simulink model "eVTOL_Small_nonandlin_algorithm_validation"  (R2024b)
settings: Solver=ode3  StartTime=0.0  StopTime=220  FixedStep=0.02  RelTol=1e-3
undefined symbols (not defined in the file): a_, b, c, c1_, deg, dttrim0, F, g, g1, h1, l1, m, MIL, PARAR, rad, rho, s, T, u_dim, ut, x_dim, xf, xmset, y_dim, yf, ymset, zf, zmset
libraries: simulink x34, aerolibconvert2 x5, aerolibwind2 x2, shared6dof x1
(part 2 of 7)

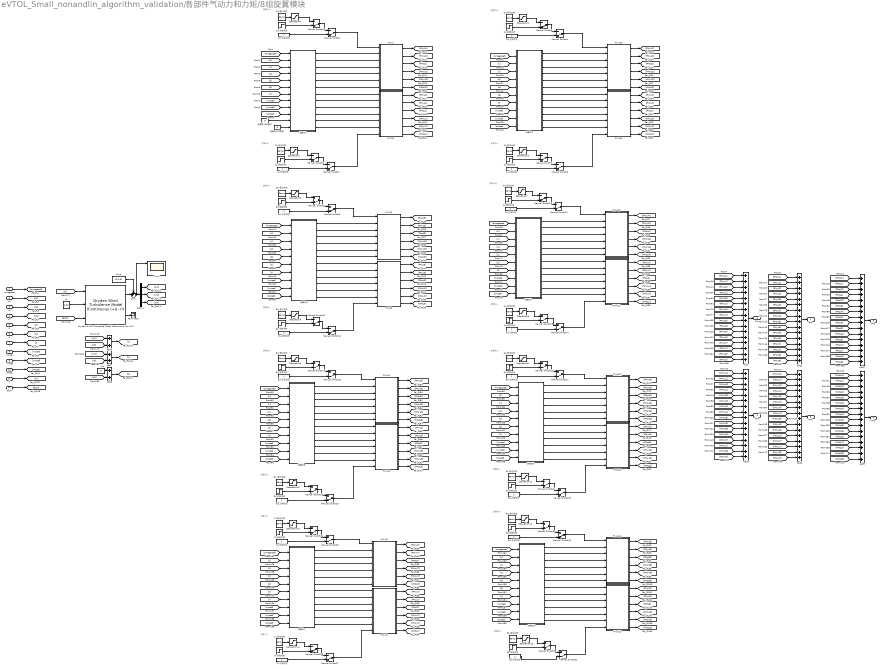
== system eVTOL_Small_nonandlin_algorithm_validation/各部件气动力和力矩/8组旋翼模块 ==
  note: 旋翼4-U
  note: 旋翼2-L
  note: 旋翼6-U
  note: 旋翼6-L
  note: 旋翼7-L
  note: 旋翼5-U
  note: 旋翼4-L
  note: 旋翼7-U
  note: 旋翼3-L
  note: 旋翼3-U
  note: 旋翼5-L
  note: 旋翼2-U
  note: 旋翼1-L
  note: 旋翼1-U
  note: 旋翼8-U
  note: 旋翼8-L
  omegaset : Inport
  u0 : Inport  Port=2
  v0 : Inport  Port=3
  w0 : Inport  Port=4
  p : Inport  Port=5
  q : Inport  Port=6
  r : Inport  Port=7
  xmset : Inport  Port=8
  ymset : Inport  Port=9
  zmset : Inport  Port=10
  H : Inport  Port=11
  DCM : Inport  Port=12
  1L-正常状态 : Constant
  1L-突发失效 : Step  Time=220  Before=1  After=0.5  SampleTime=0
  1L-退化失效 : simulink/Sources/Ramp  slope=0.3325  start=30  InitialOutput=0
  1U-正常状态 : Constant
  1U-突发失效 : Step  Time=140  Before=1  After=0.5  SampleTime=0
  1U-退化失效 : simulink/Sources/Ramp  slope=0.3325  start=30  InitialOutput=0
  2L-正常状态 : Constant
  2L-突发失效 : Step  Time=30  Before=1  After=Lp  SampleTime=0
  2L-退化失效 : simulink/Sources/Ramp  slope=0.3325  start=30  InitialOutput=0
  2U-正常状态 : Constant
  2U-突发失效 : Step  Time=80  Before=1  After=0.6  SampleTime=0
  2U-退化失效 : simulink/Sources/Ramp  slope=0.3325  start=30  InitialOutput=0
  3L-正常状态 : Constant
  3L-突发失效 : Step  Time=30  Before=1  After=Lp  SampleTime=0
  3L-退化失效 : simulink/Sources/Ramp  slope=0.3325  start=30  InitialOutput=0
  3U-正常状态 : Constant
  3U-突发失效 : Step  Time=100  Before=1  After=0.3  SampleTime=0
  3U-退化失效 : simulink/Sources/Ramp  slope=0.3325  start=30  InitialOutput=0
  4L-正常状态 : Constant
  4L-突发失效 : Step  Time=140  Before=1  After=Lp  SampleTime=0
  4L-退化失效 : simulink/Sources/Ramp  slope=0.3325  start=30  InitialOutput=0
  4U-正常状态 : Constant
  4U-突发失效 : Step  Time=160  Before=1  After=0.7  SampleTime=0
  4U-退化失效 : simulink/Sources/Ramp  slope=0.3325  start=30  InitialOutput=0
  5L -退化失效 : simulink/Sources/Ramp  slope=0.3325  start=30  InitialOutput=0
  5L-正常状态 : Constant
  5L-突发失效 : Step  Time=100  Before=1  After=Lp  SampleTime=0
  5U-正常状态 : Constant
  5U-突发失效 : Step  Time=60  Before=1  After=0.4  SampleTime=0
  5U-退化失效 : simulink/Sources/Ramp  slope=0.3325  start=30  InitialOutput=0
  6L-正常状态 : Constant
  6L-突发失效 : Step  Time=30  Before=1  After=Lp  SampleTime=0
  6L-退化失效 : simulink/Sources/Ramp  slope=0.3325  start=30  InitialOutput=0
  6U-正常状态 : Constant
  6U-突发失效 : Step  Time=160  Before=1  After=0.8  SampleTime=0
  6U-退化失效 : simulink/Sources/Ramp  slope=0.3325  start=30  InitialOutput=0
  7L-正常状态 : Constant
  7L-突发失效 : Step  Time=220  Before=1  After=0.5  SampleTime=0
  7L-退化失效 : simulink/Sources/Ramp  slope=0.3325  start=30  InitialOutput=0
  7U-正常状态 : Constant
  7U-突发失效 : Step  Time=80  Before=1  After=0.6  SampleTime=0
  7U-退化失效 : simulink/Sources/Ramp  slope=0.3325  start=30  InitialOutput=0
  8L-正常状态 : Constant
  8L-突发失效 : Step  Time=180  Before=1  After=Lp  SampleTime=0
  8L-退化失效 : simulink/Sources/Ramp  slope=0.3325  start=30  InitialOutput=0
  8U-正常状态 : Constant
  8U-突发失效 : Step  Time=180  Before=1  After=0.5  SampleTime=0
  8U-退化失效 : simulink/Sources/Ramp  slope=0.3325  start=30  InitialOutput=0
  Add{,1..5} (6 alike) : Sum  Inputs=++++++++++++++++
  Add6 : Sum
  Add7 : Sum
  Add8 : Sum
  Demux : Demux  Outputs=3
  Dryden Wind Turbulence Model (Continuous (+q +r))1 : aerolibwind2/Dryden Wind Turbulence Model  (Continuous (+q -r))  units=Metric (MKS)  spec=MIL-F-8785C  model=Continuous Dryden (+q +r)  W20=10  Wdeg=45  TurbProb=2x10^-1  L_high=1  Wingspan=1  ts=0.1  Seed=[23341 23342 23343 23344]  T_on=on
  FI-1-U : Subsystem
  FI-1-U1 : Subsystem
  FI-1-U10 : Subsystem
  FI-1-U11 : Subsystem
  FI-1-U12 : Subsystem
  FI-1-U13 : Subsystem
  FI-1-U14 : Subsystem
  FI-1-U15 : Subsystem
  FI-1-U2 : Subsystem
  FI-1-U3 : Subsystem
  FI-1-U4 : Subsystem
  FI-1-U5 : Subsystem
  FI-1-U6 : Subsystem
  FI-1-U7 : Subsystem
  FI-1-U8 : Subsystem
  FI-1-U9 : Subsystem
  Manual Switch{1..32} (32 alike) : ManualSwitch  CurrentSetting=0
  Saturation{1..16} (16 alike) : Saturate  UpperLimit=10  LowerLimit=0
  Sum : Sum  Inputs=++|
  T+W : Scope  NumInputPorts=3
  Terminator : Terminator
  Vs : Constant  Value=0.01
  Wind : Constant  Value=[0,0,0]
  wW : Constant  Value=0
  旋翼组1 : Subsystem
  旋翼组2 : Subsystem
  旋翼组3 : Subsystem
  旋翼组4 : Subsystem
  旋翼组5 : Subsystem
  旋翼组6 : Subsystem
  旋翼组7 : Subsystem
  旋翼组8 : Subsystem
  旋翼轴1前倾角° : Constant  Value=0
  旋翼轴1右倾角° : Constant  Value=0
  FMx : Outport  VectorParamsAs1DForOutWhenUnconnected=off
  FMy : Outport  Port=2  VectorParamsAs1DForOutWhenUnconnected=off
  FMz : Outport  Port=3  VectorParamsAs1DForOutWhenUnconnected=off
  MMx : Outport  Port=4  VectorParamsAs1DForOutWhenUnconnected=off
  MMy : Outport  Port=5  VectorParamsAs1DForOutWhenUnconnected=off
  MMz : Outport  Port=6  VectorParamsAs1DForOutWhenUnconnected=off
  wires:
  omegaset/1 -> [omegaset]
  u0/1 -> [u0]
  v0/1 -> [v0]
  w0/1 -> [w0]
  p/1 -> [p]
  r/1 -> [r]
  q/1 -> [q]
  xmset/1 -> [xmset]
  ymset/1 -> [ymset]
  zmset/1 -> [zmset]
  H/1 -> [H]
  DCM/1 -> [DCM]
  [v0] -> Add7/2
  [vW] -> Add7/1
  Add7/1 -> [v]
  Add6/1 -> [u]
  Demux/2 -> [vW]
  [u0] -> Add6/2
  Vs/1 -> Dryden Wind Turbulence Model (Continuous (+q +r))1/2
  Dryden Wind Turbulence Model (Continuous (+q +r))1/2 -> Terminator/1
  [uW] -> Add6/1
  Add8/1 -> [w]
  wW/1 -> Add8/1
  [w0] -> Add8/2
  Demux/3 -> [wW]
  [H] -> Dryden Wind Turbulence Model (Continuous (+q +r))1/1
  Demux/1 -> [uW]
  [DCM] -> Dryden Wind Turbulence Model (Continuous (+q +r))1/3
  [FMyL5] -> Add1/10
  [MMyU7] -> Add4/13
  [MMzU4] -> Add5/7
  [FMzU3] -> Add2/5
  [MMxU5] -> Add3/9
  [MMxL2] -> Add3/4
  [MMzU3] -> Add5/5
  [MMyU4] -> Add4/7
  [MMxU4] -> Add3/7
  旋翼轴1右倾角°/1 -> 旋翼组1/12(ILR)
  [MMzL4] -> Add5/8
  [FMyU5] -> Add1/9
  [MMxL6] -> Add3/12
  [v] -> 旋翼组2/3(v)
  [MMyL1] -> Add4/2
  [MMzU6] -> Add5/11
  [FMxU7] -> Add/13
  [FMxL6] -> Add/12
  [MMzL2] -> Add5/4
  旋翼轴1前倾角°/1 -> 旋翼组1/11(ISR)
  [MMxL5] -> Add3/10
  [MMyL5] -> Add4/10
  [FMzL7] -> Add2/14
  [omegaset] -> 旋翼组1/1(omegaset)
  [FMzU1] -> Add2/1
  [MMyU1] -> Add4/1
  [MMzU1] -> Add5/1
  [FMyL1] -> Add1/2
  [MMyU2] -> Add4/3
  [MMyU3] -> Add4/5
  [FMyU4] -> Add1/7
  [FMzL5] -> Add2/10
  [MMyU6] -> Add4/11
  [FMxL7] -> Add/14
  [MMyL6] -> Add4/12
  [FMzU6] -> Add2/11
  [FMyU1] -> Add1/1
  [zmset] -> 旋翼组1/10(zmset)
  [q] -> 旋翼组1/6(q)
  [u] -> 旋翼组1/2(u)
  [w] -> 旋翼组1/4(w)
  [FMyU6] -> Add1/11
  [MMxL3] -> Add3/6
  [p] -> 旋翼组1/5(p)
  [FMxU5] -> Add/9
  [v] -> 旋翼组1/3(v)
  [FMxL4] -> Add/8
  Add1/1 -> FMy/1
  [FMyU7] -> Add1/13
  [MMzL6] -> Add5/12
  [FMyL7] -> Add1/14
  [FMzU5] -> Add2/9
  [MMxU3] -> Add3/5
  [MMzU2] -> Add5/3
  [xmset] -> 旋翼组1/8(xmset)
  [MMyL4] -> Add4/8
  [ymset] -> 旋翼组2/9(ymset)
  [MMxL4] -> Add3/8
  [MMxU6] -> Add3/11
  [u] -> 旋翼组2/2(u)
  [MMyU5] -> Add4/9
  [omegaset] -> 旋翼组2/1(omegaset)
  [FMxU2] -> Add/3
  [q] -> 旋翼组2/6(q)
  [FMxL5] -> Add/10
  [w] -> 旋翼组2/4(w)
  [FMyL6] -> Add1/12
  [p] -> 旋翼组2/5(p)
  [FMxL8] -> Add/16
  [ymset] -> 旋翼组1/9(ymset)
  [r] -> 旋翼组1/7(r)
  Add2/1 -> FMz/1
  [FMzL6] -> Add2/12
  [FMxU8] -> Add/15
  [FMyU8] -> Add1/15
  [MMxU7] -> Add3/13
  [MMxU8] -> Add3/15
  [FMxL1] -> Add/2
  [xmset] -> 旋翼组2/8(xmset)
  [FMzU8] -> Add2/15
  [MMyL2] -> Add4/4
  [FMxU3] -> Add/5
  [zmset] -> 旋翼组2/10(zmset)
  [MMzL1] -> Add5/2
  [MMyL3] -> Add4/6
  [MMzU7] -> Add5/13
  [MMyU8] -> Add4/15
  [FMzU2] -> Add2/3
  [MMzL5] -> Add5/10
  [FMyL8] -> Add1/16
  [FMxU1] -> Add/1
  Add5/1 -> MMz/1
  Add4/1 -> MMy/1
  [MMyL7] -> Add4/14
  [MMxL1] -> Add3/2
  [MMzL7] -> Add5/14
  [MMzU5] -> Add5/9
  [FMzL2] -> Add2/4
  [FMyL2] -> Add1/4
  [MMxL8] -> Add3/16
  [FMzL4] -> Add2/8
  [MMzL3] -> Add5/6
  [MMxL7] -> Add3/14
  [MMxU1] -> Add3/1
  [FMzL3] -> Add2/6
  Add3/1 -> MMx/1
  [r] -> 旋翼组2/7(r)
  [FMyL4] -> Add1/8
  [MMyL8] -> Add4/16
  [MMxU2] -> Add3/3
  [FMzU7] -> Add2/13
  [FMxL2] -> Add/4
  [FMyU3] -> Add1/5
  [FMzL8] -> Add2/16
  Add/1 -> FMx/1
  [FMzU4] -> Add2/7
  [FMzL1] -> Add2/2
  [FMxL3] -> Add/6
  [FMyU2] -> Add1/3
  [FMxU4] -> Add/7
  [FMyL3] -> Add1/6
  [MMzU8] -> Add5/15
  [MMzL8] -> Add5/16
  [FMxU6] -> Add/11
  Sum/1 -> T+W/1, Demux/1
  Wind/1 -> Sum/1
  [zmset] -> 旋翼组6/10(zmset)
  [r] -> 旋翼组5/7(r)
  [omegaset] -> 旋翼组4/1(omegaset)
  [p] -> 旋翼组7/5(p)
  [ymset] -> 旋翼组7/9(ymset)
  [p] -> 旋翼组4/5(p)
  [omegaset] -> 旋翼组7/1(omegaset)
  [xmset] -> 旋翼组6/8(xmset)
  [w] -> 旋翼组6/4(w)
  [q] -> 旋翼组6/6(q)
  [xmset] -> 旋翼组7/8(xmset)
  [zmset] -> 旋翼组8/10(zmset)
  [omegaset] -> 旋翼组6/1(omegaset)
  [v] -> 旋翼组5/3(v)
  [v] -> 旋翼组6/3(v)
  [q] -> 旋翼组7/6(q)
  [p] -> 旋翼组6/5(p)
  [ymset] -> 旋翼组8/9(ymset)
  [r] -> 旋翼组7/7(r)
  [p] -> 旋翼组8/5(p)
  [xmset] -> 旋翼组4/8(xmset)
  [w] -> 旋翼组4/4(w)
  [u] -> 旋翼组8/2(u)
  [q] -> 旋翼组4/6(q)
  [omegaset] -> 旋翼组8/1(omegaset)
  [u] -> 旋翼组6/2(u)
  [zmset] -> 旋翼组3/10(zmset)
  [ymset] -> 旋翼组5/9(ymset)
  [u] -> 旋翼组3/2(u)
  [u] -> 旋翼组4/2(u)
  [r] -> 旋翼组6/7(r)
  [w] -> 旋翼组3/4(w)
  [zmset] -> 旋翼组4/10(zmset)
  [q] -> 旋翼组3/6(q)
  [ymset] -> 旋翼组4/9(ymset)
  [xmset] -> 旋翼组3/8(xmset)
  [p] -> 旋翼组3/5(p)
  [r] -> 旋翼组8/7(r)
  [v] -> 旋翼组8/3(v)
  [q] -> 旋翼组5/6(q)
  [p] -> 旋翼组5/5(p)
  [ymset] -> 旋翼组3/9(ymset)
  [r] -> 旋翼组3/7(r)
  [u] -> 旋翼组5/2(u)
  [r] -> 旋翼组4/7(r)
  [v] -> 旋翼组4/3(v)
  [v] -> 旋翼组7/3(v)
  [ymset] -> 旋翼组6/9(ymset)
  [xmset] -> 旋翼组5/8(xmset)
  [w] -> 旋翼组7/4(w)
  [xmset] -> 旋翼组8/8(xmset)
  [v] -> 旋翼组3/3(v)
  [q] -> 旋翼组8/6(q)
  [zmset] -> 旋翼组7/10(zmset)
  [w] -> 旋翼组8/4(w)
  [u] -> 旋翼组7/2(u)
  [zmset] -> 旋翼组5/10(zmset)
  [w] -> 旋翼组5/4(w)
  [omegaset] -> 旋翼组3/1(omegaset)
  [omegaset] -> 旋翼组5/1(omegaset)
  Dryden Wind Turbulence Model (Continuous (+q +r))1/1 -> Sum/2
  旋翼组1/1(FMxU1) -> FI-1-U/2(FMxU1)
  旋翼组1/2(FMyU1) -> FI-1-U/3(FMyU1)
  旋翼组1/3(FMzU1) -> FI-1-U/4(FMzU1)
  旋翼组1/4(MMxU1) -> FI-1-U/5(MMxU1)
  旋翼组1/5(MMyU1) -> FI-1-U/6(MMyU1)
  旋翼组1/6(MMzU1) -> FI-1-U/7(MMzU1)
  FI-1-U/6(Out6) -> [MMzU1]
  FI-1-U/5(Out5) -> [MMyU1]
  FI-1-U/4(Out4) -> [MMxU1]
  FI-1-U/3(Out3) -> [FMzU1]
  FI-1-U/2(Out2) -> [FMyU1]
  FI-1-U/1(Out1) -> [FMxU1]
  FI-1-U2/3(Out3) -> [FMzU3]
  FI-1-U2/6(Out6) -> [MMzU3]
  FI-1-U2/1(Out1) -> [FMxU3]
  FI-1-U3/1(Out1) -> [FMxL3]
  FI-1-U2/2(Out2) -> [FMyU3]
  FI-1-U3/2(Out2) -> [FMyL3]
  FI-1-U2/5(Out5) -> [MMyU3]
  FI-1-U2/4(Out4) -> [MMxU3]
  FI-1-U3/4(Out4) -> [MMxL3]
  FI-1-U3/5(Out5) -> [MMyL3]
  FI-1-U3/3(Out3) -> [FMzL3]
  5U-突发失效/1 -> Manual Switch17/2
  3L-退化失效/1 -> Saturation6/1
  Manual Switch11/1 -> Manual Switch10/1
  6U-正常状态/1 -> Manual Switch21/2
  3L-正常状态/1 -> Manual Switch10/2
  1U-突发失效/1 -> Manual Switch20/2
  4U-正常状态/1 -> Manual Switch12/2
  2U-正常状态/1 -> Manual Switch4/2
  5L-正常状态/1 -> Manual Switch18/2
  Saturation12/1 -> Manual Switch24/1
  7U-退化失效/1 -> Saturation13/1
  Saturation6/1 -> Manual Switch11/1
  4L-退化失效/1 -> Saturation8/1
  Manual Switch20/1 -> Manual Switch1/1
  4L-突发失效/1 -> Manual Switch15/2
  Saturation14/1 -> Manual Switch28/1
  7L-退化失效/1 -> Saturation14/1
  6L-退化失效/1 -> Saturation12/1
  4U-退化失效/1 -> Saturation7/1
  6U-突发失效/1 -> Manual Switch22/2
  Saturation10/1 -> Manual Switch19/1
  Manual Switch28/1 -> Manual Switch27/1
  6L-突发失效/1 -> Manual Switch24/2
  4U-突发失效/1 -> Manual Switch13/2
  Saturation7/1 -> Manual Switch13/1
  Manual Switch13/1 -> Manual Switch12/1
  Manual Switch7/1 -> Manual Switch6/1
  1L-突发失效/1 -> Manual Switch3/2
  7L-正常状态/1 -> Manual Switch27/2
  Saturation13/1 -> Manual Switch26/1
  1L-正常状态/1 -> Manual Switch2/2
  Manual Switch26/1 -> Manual Switch25/1
  1U-退化失效/1 -> Saturation4/1
  Manual Switch9/1 -> Manual Switch8/1
  Manual Switch3/1 -> Manual Switch2/1
  Manual Switch5/1 -> Manual Switch4/1
  2U-突发失效/1 -> Manual Switch5/2
  Manual Switch22/1 -> Manual Switch21/1
  2U-退化失效/1 -> Saturation2/1
  1U-正常状态/1 -> Manual Switch1/2
  Saturation2/1 -> Manual Switch5/1
  2L-突发失效/1 -> Manual Switch7/2
  3U-突发失效/1 -> Manual Switch9/2
  Manual Switch15/1 -> Manual Switch14/1
  4L-正常状态/1 -> Manual Switch14/2
  Saturation8/1 -> Manual Switch15/1
  3U-正常状态/1 -> Manual Switch8/2
  Manual Switch17/1 -> Manual Switch16/1
  5U-退化失效/1 -> Saturation9/1
  1L-退化失效/1 -> Saturation1/1
  5U-正常状态/1 -> Manual Switch16/2
  5L -退化失效/1 -> Saturation10/1
  2L-退化失效/1 -> Saturation3/1
  Saturation11/1 -> Manual Switch22/1
  Manual Switch19/1 -> Manual Switch18/1
  Saturation9/1 -> Manual Switch17/1
  2L-正常状态/1 -> Manual Switch6/2
  Saturation3/1 -> Manual Switch7/1
  Saturation5/1 -> Manual Switch9/1
  6U-退化失效/1 -> Saturation11/1
  Manual Switch24/1 -> Manual Switch23/1
  3L-突发失效/1 -> Manual Switch11/2
  7U-突发失效/1 -> Manual Switch26/2
  5L-突发失效/1 -> Manual Switch19/2
  6L-正常状态/1 -> Manual Switch23/2
  Saturation1/1 -> Manual Switch3/1
  3U-退化失效/1 -> Saturation5/1
  Saturation4/1 -> Manual Switch20/1
  7U-正常状态/1 -> Manual Switch25/2
  7L-突发失效/1 -> Manual Switch28/2
  Manual Switch1/1 -> FI-1-U/1(Fault inject)
  旋翼组1/7(FMxL1) -> FI-1-U1/1(FMxU1)
  旋翼组1/8(FMyL1) -> FI-1-U1/2(FMyU1)
  旋翼组1/9(FMzL1) -> FI-1-U1/3(FMzU1)
  旋翼组1/10(MMxL1) -> FI-1-U1/4(MMxU1)
  旋翼组1/11(MMyL1) -> FI-1-U1/5(MMyU1)
  旋翼组1/12(MMzL1) -> FI-1-U1/6(MMzU1)
  FI-1-U1/1(Out1) -> [FMxL1]
  FI-1-U1/2(Out2) -> [FMyL1]
  FI-1-U1/3(Out3) -> [FMzL1]
  FI-1-U1/4(Out4) -> [MMxL1]
  FI-1-U1/5(Out5) -> [MMyL1]
  FI-1-U1/6(Out6) -> [MMzL1]
  Manual Switch2/1 -> FI-1-U1/7(Fault inject)
  旋翼组3/5(MMyU3) -> FI-1-U2/6(MMyU1)
  旋翼组3/6(MMzU3) -> FI-1-U2/7(MMzU1)
  Manual Switch8/1 -> FI-1-U2/1(Fault inject)
  旋翼组3/7(FMxL3) -> FI-1-U3/1(FMxU1)
  旋翼组3/10(MMxL3) -> FI-1-U3/4(MMxU1)
  旋翼组3/1(FMxU3) -> FI-1-U2/2(FMxU1)
  旋翼组3/9(FMzL3) -> FI-1-U3/3(FMzU1)
  旋翼组3/4(MMxU3) -> FI-1-U2/5(MMxU1)
  旋翼组3/12(MMzL3) -> FI-1-U3/6(MMzU1)
  旋翼组3/2(FMyU3) -> FI-1-U2/3(FMyU1)
  Manual Switch10/1 -> FI-1-U3/7(Fault inject)
  旋翼组3/8(FMyL3) -> FI-1-U3/2(FMyU1)
  旋翼组3/3(FMzU3) -> FI-1-U2/4(FMzU1)
  旋翼组3/11(MMyL3) -> FI-1-U3/5(MMyU1)
  FI-1-U3/6(Out6) -> [MMzL3]
  FI-1-U5/6(Out6) -> [MMzL5]
  旋翼组5/11(MMyL5) -> FI-1-U5/5(MMyU1)
  旋翼组5/3(FMzU5) -> FI-1-U4/4(FMzU1)
  Manual Switch16/1 -> FI-1-U4/1(Fault inject)
  旋翼组5/10(MMxL5) -> FI-1-U5/4(MMxU1)
  FI-1-U4/2(Out2) -> [FMyU5]
  FI-1-U4/5(Out5) -> [MMyU5]
  旋翼组5/7(FMxL5) -> FI-1-U5/1(FMxU1)
  旋翼组5/5(MMyU5) -> FI-1-U4/6(MMyU1)
  旋翼组5/8(FMyL5) -> FI-1-U5/2(FMyU1)
  旋翼组5/9(FMzL5) -> FI-1-U5/3(FMzU1)
  Manual Switch18/1 -> FI-1-U5/7(Fault inject)
  FI-1-U4/6(Out6) -> [MMzU5]
  旋翼组5/2(FMyU5) -> FI-1-U4/3(FMyU1)
  FI-1-U5/4(Out4) -> [MMxL5]
  旋翼组5/4(MMxU5) -> FI-1-U4/5(MMxU1)
  旋翼组5/6(MMzU5) -> FI-1-U4/7(MMzU1)
  FI-1-U4/1(Out1) -> [FMxU5]
  FI-1-U4/3(Out3) -> [FMzU5]
  FI-1-U5/3(Out3) -> [FMzL5]
  旋翼组5/12(MMzL5) -> FI-1-U5/6(MMzU1)
  旋翼组5/1(FMxU5) -> FI-1-U4/2(FMxU1)
  FI-1-U5/5(Out5) -> [MMyL5]
  FI-1-U5/1(Out1) -> [FMxL5]
  FI-1-U5/2(Out2) -> [FMyL5]
  FI-1-U4/4(Out4) -> [MMxU5]
  旋翼组7/7(FMxL7) -> FI-1-U7/1(FMxU1)
  旋翼组7/4(MMxU7) -> FI-1-U6/5(MMxU1)
  Manual Switch27/1 -> FI-1-U7/7(Fault inject)
  旋翼组7/1(FMxU7) -> FI-1-U6/2(FMxU1)
  Manual Switch25/1 -> FI-1-U6/1(Fault inject)
  旋翼组7/8(FMyL7) -> FI-1-U7/2(FMyU1)
  旋翼组7/11(MMyL7) -> FI-1-U7/5(MMyU1)
  旋翼组7/9(FMzL7) -> FI-1-U7/3(FMzU1)
  旋翼组7/10(MMxL7) -> FI-1-U7/4(MMxU1)
  FI-1-U6/2(Out2) -> [FMyU7]
  旋翼组7/3(FMzU7) -> FI-1-U6/4(FMzU1)
  旋翼组7/6(MMzU7) -> FI-1-U6/7(MMzU1)
  旋翼组7/5(MMyU7) -> FI-1-U6/6(MMyU1)
  FI-1-U6/6(Out6) -> [MMzU7]
  旋翼组7/12(MMzL7) -> FI-1-U7/6(MMzU1)
  FI-1-U7/6(Out6) -> [MMzL7]
  旋翼组7/2(FMyU7) -> FI-1-U6/3(FMyU1)
  FI-1-U6/3(Out3) -> [FMzU7]
  FI-1-U6/4(Out4) -> [MMxU7]
  FI-1-U7/1(Out1) -> [FMxL7]
  FI-1-U6/5(Out5) -> [MMyU7]
  FI-1-U7/2(Out2) -> [FMyL7]
  FI-1-U7/5(Out5) -> [MMyL7]
  FI-1-U6/1(Out1) -> [FMxU7]
  FI-1-U7/3(Out3) -> [FMzL7]
  FI-1-U7/4(Out4) -> [MMxL7]
  旋翼组2/4(MMxU2) -> FI-1-U8/5(MMxU1)
  FI-1-U8/1(Out1) -> [FMxU2]
  FI-1-U8/6(Out6) -> [MMzU2]
  FI-1-U9/5(Out5) -> [MMyL2]
  FI-1-U9/2(Out2) -> [FMyL2]
  Manual Switch4/1 -> FI-1-U8/1(Fault inject)
  旋翼组2/2(FMyU2) -> FI-1-U8/3(FMyU1)
  旋翼组2/7(FMxL2) -> FI-1-U9/1(FMxU1)
  旋翼组2/10(MMxL2) -> FI-1-U9/4(MMxU1)
  FI-1-U8/2(Out2) -> [FMyU2]
  FI-1-U8/4(Out4) -> [MMxU2]
  FI-1-U9/4(Out4) -> [MMxL2]
  旋翼组2/3(FMzU2) -> FI-1-U8/4(FMzU1)
  旋翼组2/5(MMyU2) -> FI-1-U8/6(MMyU1)
  旋翼组2/1(FMxU2) -> FI-1-U8/2(FMxU1)
  旋翼组2/9(FMzL2) -> FI-1-U9/3(FMzU1)
  旋翼组2/8(FMyL2) -> FI-1-U9/2(FMyU1)
  旋翼组2/6(MMzU2) -> FI-1-U8/7(MMzU1)
  FI-1-U8/5(Out5) -> [MMyU2]
  旋翼组2/11(MMyL2) -> FI-1-U9/5(MMyU1)
  旋翼组2/12(MMzL2) -> FI-1-U9/6(MMzU1)
  FI-1-U8/3(Out3) -> [FMzU2]
  FI-1-U9/1(Out1) -> [FMxL2]
  FI-1-U9/6(Out6) -> [MMzL2]
  FI-1-U9/3(Out3) -> [FMzL2]
  Manual Switch6/1 -> FI-1-U9/7(Fault inject)
  旋翼组4/2(FMyU4) -> FI-1-U10/3(FMyU1)
  旋翼组4/11(MMyL4) -> FI-1-U11/5(MMyU1)
  旋翼组4/6(MMzU4) -> FI-1-U10/7(MMzU1)
  旋翼组4/4(MMxU4) -> FI-1-U10/5(MMxU1)
  FI-1-U10/3(Out3) -> [FMzU4]
  FI-1-U11/6(Out6) -> [MMzL4]
  旋翼组4/9(FMzL4) -> FI-1-U11/3(FMzU1)
  旋翼组4/3(FMzU4) -> FI-1-U10/4(FMzU1)
  旋翼组4/7(FMxL4) -> FI-1-U11/1(FMxU1)
  旋翼组4/12(MMzL4) -> FI-1-U11/6(MMzU1)
  旋翼组4/1(FMxU4) -> FI-1-U10/2(FMxU1)
  FI-1-U10/4(Out4) -> [MMxU4]
  旋翼组4/5(MMyU4) -> FI-1-U10/6(MMyU1)
  旋翼组4/10(MMxL4) -> FI-1-U11/4(MMxU1)
  旋翼组4/8(FMyL4) -> FI-1-U11/2(FMyU1)
  Manual Switch14/1 -> FI-1-U11/7(Fault inject)
  Manual Switch12/1 -> FI-1-U10/1(Fault inject)
  FI-1-U10/6(Out6) -> [MMzU4]
  FI-1-U11/2(Out2) -> [FMyL4]
  FI-1-U10/5(Out5) -> [MMyU4]
  FI-1-U10/2(Out2) -> [FMyU4]
  FI-1-U10/1(Out1) -> [FMxU4]
  FI-1-U11/5(Out5) -> [MMyL4]
  FI-1-U11/4(Out4) -> [MMxL4]
  FI-1-U11/3(Out3) -> [FMzL4]
  FI-1-U11/1(Out1) -> [FMxL4]
  旋翼组6/9(FMzL6) -> FI-1-U13/3(FMzU1)
  旋翼组6/4(MMxU6) -> FI-1-U12/5(MMxU1)
  FI-1-U12/1(Out1) -> [FMxU6]
  FI-1-U12/2(Out2) -> [FMyU6]
  FI-1-U13/4(Out4) -> [MMxL6]
  FI-1-U13/2(Out2) -> [FMyL6]
  Manual Switch21/1 -> FI-1-U12/1(Fault inject)
  旋翼组6/5(MMyU6) -> FI-1-U12/6(MMyU1)
  FI-1-U12/6(Out6) -> [MMzU6]
  旋翼组6/1(FMxU6) -> FI-1-U12/2(FMxU1)
  旋翼组6/12(MMzL6) -> FI-1-U13/6(MMzU1)
  旋翼组6/2(FMyU6) -> FI-1-U12/3(FMyU1)
  FI-1-U13/6(Out6) -> [MMzL6]
  旋翼组6/6(MMzU6) -> FI-1-U12/7(MMzU1)
  旋翼组6/11(MMyL6) -> FI-1-U13/5(MMyU1)
  FI-1-U12/3(Out3) -> [FMzU6]
  旋翼组6/3(FMzU6) -> FI-1-U12/4(FMzU1)
  旋翼组6/8(FMyL6) -> FI-1-U13/2(FMyU1)
  旋翼组6/7(FMxL6) -> FI-1-U13/1(FMxU1)
  FI-1-U13/1(Out1) -> [FMxL6]
  FI-1-U12/5(Out5) -> [MMyU6]
  FI-1-U12/4(Out4) -> [MMxU6]
  旋翼组6/10(MMxL6) -> FI-1-U13/4(MMxU1)
  Manual Switch23/1 -> FI-1-U13/7(Fault inject)
  FI-1-U13/3(Out3) -> [FMzL6]
  FI-1-U13/5(Out5) -> [MMyL6]
  旋翼组8/10(MMxL8) -> FI-1-U15/4(MMxU1)
  旋翼组8/4(MMxU8) -> FI-1-U14/5(MMxU1)
  FI-1-U15/4(Out4) -> [MMxL8]
  FI-1-U15/6(Out6) -> [MMzL8]
  FI-1-U14/6(Out6) -> [MMzU8]
  FI-1-U15/3(Out3) -> [FMzL8]
  Manual Switch29/1 -> FI-1-U14/1(Fault inject)
  FI-1-U14/2(Out2) -> [FMyU8]
  Manual Switch31/1 -> FI-1-U15/7(Fault inject)
  旋翼组8/5(MMyU8) -> FI-1-U14/6(MMyU1)
  旋翼组8/3(FMzU8) -> FI-1-U14/4(FMzU1)
  旋翼组8/6(MMzU8) -> FI-1-U14/7(MMzU1)
  旋翼组8/1(FMxU8) -> FI-1-U14/2(FMxU1)
  FI-1-U14/4(Out4) -> [MMxU8]
  FI-1-U14/5(Out5) -> [MMyU8]
  旋翼组8/9(FMzL8) -> FI-1-U15/3(FMzU1)
  旋翼组8/2(FMyU8) -> FI-1-U14/3(FMyU1)
  FI-1-U15/1(Out1) -> [FMxL8]
  FI-1-U14/1(Out1) -> [FMxU8]
  FI-1-U14/3(Out3) -> [FMzU8]
  旋翼组8/11(MMyL8) -> FI-1-U15/5(MMyU1)
  旋翼组8/12(MMzL8) -> FI-1-U15/6(MMzU1)
  旋翼组8/7(FMxL8) -> FI-1-U15/1(FMxU1)
  旋翼组8/8(FMyL8) -> FI-1-U15/2(FMyU1)
  FI-1-U15/2(Out2) -> [FMyL8]
  Manual Switch30/1 -> Manual Switch29/1
  8U-退化失效/1 -> Saturation15/1
  Manual Switch32/1 -> Manual Switch31/1
  8L-正常状态/1 -> Manual Switch31/2
  8L-退化失效/1 -> Saturation16/1
  8L-突发失效/1 -> Manual Switch32/2
  8U-突发失效/1 -> Manual Switch30/2
  8U-正常状态/1 -> Manual Switch29/2
  Saturation16/1 -> Manual Switch32/1
  Saturation15/1 -> Manual Switch30/1
  FI-1-U15/5(Out5) -> [MMyL8]

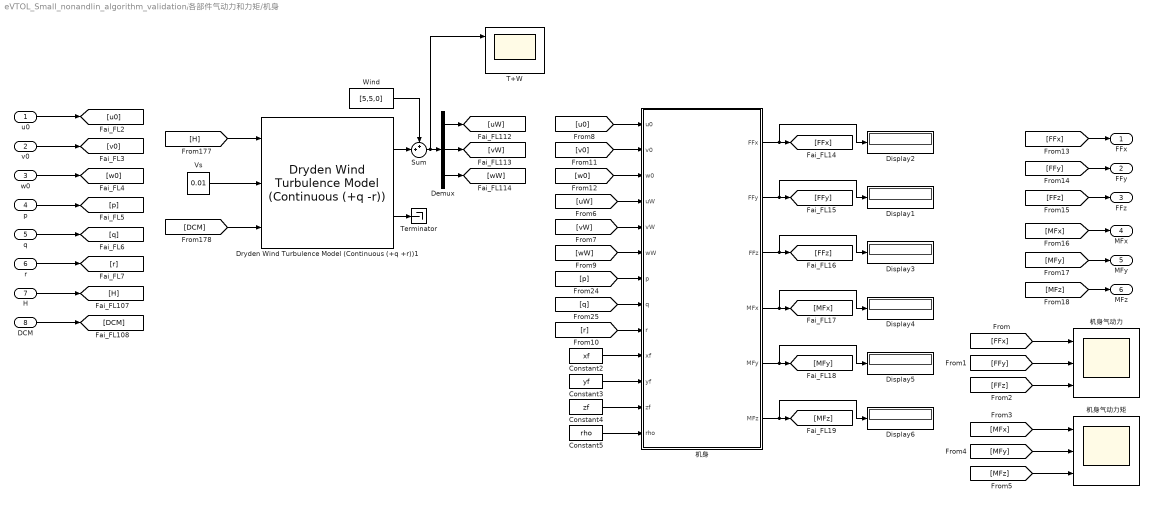
== system eVTOL_Small_nonandlin_algorithm_validation/各部件气动力和力矩/机身 ==
  "u0 " : Inport
  v0 : Inport  Port=2
  w0 : Inport  Port=3
  p : Inport  Port=4
  q : Inport  Port=5
  r : Inport  Port=6
  H : Inport  Port=7
  DCM : Inport  Port=8
  Constant2 : Constant  Value=xf
  Constant3 : Constant  Value=yf
  Constant4 : Constant  Value=zf
  Constant5 : Constant  Value=rho
  Demux : Demux  Outputs=3
  Display{1..6} (6 alike) : Display
  Dryden Wind Turbulence Model (Continuous (+q +r))1 : aerolibwind2/Dryden Wind Turbulence Model  (Continuous (+q -r))  units=Metric (MKS)  spec=MIL-F-8785C  model=Continuous Dryden (+q +r)  W20=10  Wdeg=45  TurbProb=2x10^-1  L_high=1  Wingspan=1  ts=0.1  Seed=[23341 23342 23343 23344]  T_on=on
  Sum : Sum  Inputs=++|
  T+W : Scope  NumInputPorts=3
  Terminator : Terminator
  Vs : Constant  Value=0.01
  Wind : Constant  Value=[5,5,0]  VectorParams1D=off
  机身 : MATLAB Function  TreatAsAtomicUnit=on
  机身气动力 : Scope  NumInputPorts=3
  机身气动力矩 : Scope  NumInputPorts=3
  FFx : Outport  VectorParamsAs1DForOutWhenUnconnected=off
  FFy : Outport  Port=2  VectorParamsAs1DForOutWhenUnconnected=off
  FFz : Outport  Port=3  VectorParamsAs1DForOutWhenUnconnected=off
  MFx : Outport  Port=4  VectorParamsAs1DForOutWhenUnconnected=off
  MFy : Outport  Port=5  VectorParamsAs1DForOutWhenUnconnected=off
  MFz : Outport  Port=6  VectorParamsAs1DForOutWhenUnconnected=off
  wires:
  [v0] -> 机身/2(v0)
  [u0] -> 机身/1(u0)
  [w0] -> 机身/3(w0)
  Constant3/1 -> 机身/11(yf)
  机身/5(MFy) -> Display5/1, [MFy]
  Constant4/1 -> 机身/12(zf)
  [r] -> 机身/9(r)
  [p] -> 机身/7(p)
  机身/2(FFy) -> Display1/1, [FFy]
  机身/1(FFx) -> Display2/1, [FFx]
  Constant5/1 -> 机身/13(rho)
  机身/3(FFz) -> Display3/1, [FFz]
  Constant2/1 -> 机身/10(xf)
  机身/6(MFz) -> Display6/1, [MFz]
  机身/4(MFx) -> Display4/1, [MFx]
  [q] -> 机身/8(q)
  v0/1 -> [v0]
  "u0 "/1 -> [u0]
  w0/1 -> [w0]
  p/1 -> [p]
  r/1 -> [r]
  q/1 -> [q]
  Demux/1 -> [uW]
  [H] -> Dryden Wind Turbulence Model (Continuous (+q +r))1/1
  Dryden Wind Turbulence Model (Continuous (+q +r))1/2 -> Terminator/1
  Demux/2 -> [vW]
  Demux/3 -> [wW]
  [DCM] -> Dryden Wind Turbulence Model (Continuous (+q +r))1/3
  Vs/1 -> Dryden Wind Turbulence Model (Continuous (+q +r))1/2
  DCM/1 -> [DCM]
  H/1 -> [H]
  [uW] -> 机身/4(uW)
  [vW] -> 机身/5(vW)
  [wW] -> 机身/6(wW)
  [FFx] -> FFx/1
  [FFy] -> FFy/1
  [FFz] -> FFz/1
  [MFx] -> MFx/1
  [MFy] -> MFy/1
  [MFz] -> MFz/1
  [FFx] -> 机身气动力/1
  [FFy] -> 机身气动力/2
  [FFz] -> 机身气动力/3
  [MFx] -> 机身气动力矩/1
  [MFy] -> 机身气动力矩/2
  [MFz] -> 机身气动力矩/3
  Sum/1 -> T+W/1, Demux/1
  Wind/1 -> Sum/1
  Dryden Wind Turbulence Model (Continuous (+q +r))1/1 -> Sum/2

== system eVTOL_Small_nonandlin_algorithm_validation/Subsystem1/Subsystem1/Subsystem ==
  ut : Inport
  y : Inport  Port=2
  Clock : Clock
  Constant : Constant  Value=y_dim
  Constant1 : Constant  Value=c
  Constant2 : Constant  Value=b
  Derivative : Derivative
  MATLAB Function : MATLAB Function  TreatAsAtomicUnit=on
  Signal Specification : SignalSpecification  Dimensions=[y_dim,1]
  Signal Specification1 : SignalSpecification  Dimensions=[u_dim,1]
  Signal Specification2 : SignalSpecification  Dimensions=[y_dim*2,1]
  y_ : Outport
  wires:
  ut/1 -> Signal Specification1/1
  Derivative/1 -> MATLAB Function/2(dy)
  Clock/1 -> MATLAB Function/4(t)
  Constant/1 -> MATLAB Function/5(y_dim)
  Constant1/1 -> MATLAB Function/6(c)
  Constant2/1 -> MATLAB Function/7(b)
  Signal Specification/1 -> MATLAB Function/1(y), Derivative/1
  y/1 -> Signal Specification/1
  Signal Specification1/1 -> MATLAB Function/3(u)
  MATLAB Function/1(y_) -> Signal Specification2/1
  Signal Specification2/1 -> y_/1

== system eVTOL_Small_nonandlin_algorithm_validation/各部件气动力和力矩/8组旋翼模块/FI-1-U ==
  Fault inject : Inport
  FMxU1 : Inport  Port=2
  FMyU1 : Inport  Port=3
  FMzU1 : Inport  Port=4
  MMxU1 : Inport  Port=5
  MMyU1 : Inport  Port=6
  MMzU1 : Inport  Port=7
  Product{,1..5} (6 alike) : Product
  Out1 : Outport
  Out2 : Outport  Port=2
  Out3 : Outport  Port=3
  Out4 : Outport  Port=4
  Out5 : Outport  Port=5
  Out6 : Outport  Port=6
  wires:
  FMxU1/1 -> Product/2
  FMyU1/1 -> Product1/2
  FMzU1/1 -> Product2/2
  MMxU1/1 -> Product3/2
  MMyU1/1 -> Product4/2
  MMzU1/1 -> Product5/2
  Product/1 -> Out1/1
  Product1/1 -> Out2/1
  Product2/1 -> Out3/1
  Product3/1 -> Out4/1
  Product4/1 -> Out5/1
  Product5/1 -> Out6/1
  Fault inject/1 -> Product5/1, Product4/1, Product3/1, Product2/1, Product1/1, Product/1

== system eVTOL_Small_nonandlin_algorithm_validation/各部件气动力和力矩/8组旋翼模块/FI-1-U1 ==
  FMxU1 : Inport
  FMyU1 : Inport  Port=2
  FMzU1 : Inport  Port=3
  MMxU1 : Inport  Port=4
  MMyU1 : Inport  Port=5
  MMzU1 : Inport  Port=6
  Fault inject : Inport  Port=7
  Product{,1..5} (6 alike) : Product
  Out1 : Outport
  Out2 : Outport  Port=2
  Out3 : Outport  Port=3
  Out4 : Outport  Port=4
  Out5 : Outport  Port=5
  Out6 : Outport  Port=6
  wires:
  FMxU1/1 -> Product/2
  FMyU1/1 -> Product1/2
  FMzU1/1 -> Product2/2
  MMxU1/1 -> Product3/2
  MMyU1/1 -> Product4/2
  MMzU1/1 -> Product5/2
  Product/1 -> Out1/1
  Product1/1 -> Out2/1
  Product2/1 -> Out3/1
  Product3/1 -> Out4/1
  Product4/1 -> Out5/1
  Product5/1 -> Out6/1
  Fault inject/1 -> Product5/1, Product4/1, Product3/1, Product2/1, Product1/1, Product/1

== system eVTOL_Small_nonandlin_algorithm_validation/各部件气动力和力矩/8组旋翼模块/FI-1-U10 ==
  Fault inject : Inport
  FMxU1 : Inport  Port=2
  FMyU1 : Inport  Port=3
  FMzU1 : Inport  Port=4
  MMxU1 : Inport  Port=5
  MMyU1 : Inport  Port=6
  MMzU1 : Inport  Port=7
  Product{,1..5} (6 alike) : Product
  Out1 : Outport
  Out2 : Outport  Port=2
  Out3 : Outport  Port=3
  Out4 : Outport  Port=4
  Out5 : Outport  Port=5
  Out6 : Outport  Port=6
  wires:
  FMxU1/1 -> Product/2
  FMyU1/1 -> Product1/2
  FMzU1/1 -> Product2/2
  MMxU1/1 -> Product3/2
  MMyU1/1 -> Product4/2
  MMzU1/1 -> Product5/2
  Product/1 -> Out1/1
  Product1/1 -> Out2/1
  Product2/1 -> Out3/1
  Product3/1 -> Out4/1
  Product4/1 -> Out5/1
  Product5/1 -> Out6/1
  Fault inject/1 -> Product5/1, Product4/1, Product3/1, Product2/1, Product1/1, Product/1

== system eVTOL_Small_nonandlin_algorithm_validation/各部件气动力和力矩/8组旋翼模块/FI-1-U11 ==
  FMxU1 : Inport
  FMyU1 : Inport  Port=2
  FMzU1 : Inport  Port=3
  MMxU1 : Inport  Port=4
  MMyU1 : Inport  Port=5
  MMzU1 : Inport  Port=6
  Fault inject : Inport  Port=7
  Product{,1..5} (6 alike) : Product
  Out1 : Outport
  Out2 : Outport  Port=2
  Out3 : Outport  Port=3
  Out4 : Outport  Port=4
  Out5 : Outport  Port=5
  Out6 : Outport  Port=6
  wires:
  FMxU1/1 -> Product/2
  FMyU1/1 -> Product1/2
  FMzU1/1 -> Product2/2
  MMxU1/1 -> Product3/2
  MMyU1/1 -> Product4/2
  MMzU1/1 -> Product5/2
  Product/1 -> Out1/1
  Product1/1 -> Out2/1
  Product2/1 -> Out3/1
  Product3/1 -> Out4/1
  Product4/1 -> Out5/1
  Product5/1 -> Out6/1
  Fault inject/1 -> Product5/1, Product4/1, Product3/1, Product2/1, Product1/1, Product/1

== system eVTOL_Small_nonandlin_algorithm_validation/各部件气动力和力矩/8组旋翼模块/FI-1-U12 ==
  Fault inject : Inport
  FMxU1 : Inport  Port=2
  FMyU1 : Inport  Port=3
  FMzU1 : Inport  Port=4
  MMxU1 : Inport  Port=5
  MMyU1 : Inport  Port=6
  MMzU1 : Inport  Port=7
  Product{,1..5} (6 alike) : Product
  Out1 : Outport
  Out2 : Outport  Port=2
  Out3 : Outport  Port=3
  Out4 : Outport  Port=4
  Out5 : Outport  Port=5
  Out6 : Outport  Port=6
  wires:
  FMxU1/1 -> Product/2
  FMyU1/1 -> Product1/2
  FMzU1/1 -> Product2/2
  MMxU1/1 -> Product3/2
  MMyU1/1 -> Product4/2
  MMzU1/1 -> Product5/2
  Product/1 -> Out1/1
  Product1/1 -> Out2/1
  Product2/1 -> Out3/1
  Product3/1 -> Out4/1
  Product4/1 -> Out5/1
  Product5/1 -> Out6/1
  Fault inject/1 -> Product5/1, Product4/1, Product3/1, Product2/1, Product1/1, Product/1

== system eVTOL_Small_nonandlin_algorithm_validation/各部件气动力和力矩/8组旋翼模块/FI-1-U13 ==
  FMxU1 : Inport
  FMyU1 : Inport  Port=2
  FMzU1 : Inport  Port=3
  MMxU1 : Inport  Port=4
  MMyU1 : Inport  Port=5
  MMzU1 : Inport  Port=6
  Fault inject : Inport  Port=7
  Product{,1..5} (6 alike) : Product
  Out1 : Outport
  Out2 : Outport  Port=2
  Out3 : Outport  Port=3
  Out4 : Outport  Port=4
  Out5 : Outport  Port=5
  Out6 : Outport  Port=6
  wires:
  FMxU1/1 -> Product/2
  FMyU1/1 -> Product1/2
  FMzU1/1 -> Product2/2
  MMxU1/1 -> Product3/2
  MMyU1/1 -> Product4/2
  MMzU1/1 -> Product5/2
  Product/1 -> Out1/1
  Product1/1 -> Out2/1
  Product2/1 -> Out3/1
  Product3/1 -> Out4/1
  Product4/1 -> Out5/1
  Product5/1 -> Out6/1
  Fault inject/1 -> Product5/1, Product4/1, Product3/1, Product2/1, Product1/1, Product/1

== system eVTOL_Small_nonandlin_algorithm_validation/各部件气动力和力矩/8组旋翼模块/FI-1-U14 ==
  Fault inject : Inport
  FMxU1 : Inport  Port=2
  FMyU1 : Inport  Port=3
  FMzU1 : Inport  Port=4
  MMxU1 : Inport  Port=5
  MMyU1 : Inport  Port=6
  MMzU1 : Inport  Port=7
  Product{,1..5} (6 alike) : Product
  Out1 : Outport
  Out2 : Outport  Port=2
  Out3 : Outport  Port=3
  Out4 : Outport  Port=4
  Out5 : Outport  Port=5
  Out6 : Outport  Port=6
  wires:
  FMxU1/1 -> Product/2
  FMyU1/1 -> Product1/2
  FMzU1/1 -> Product2/2
  MMxU1/1 -> Product3/2
  MMyU1/1 -> Product4/2
  MMzU1/1 -> Product5/2
  Product/1 -> Out1/1
  Product1/1 -> Out2/1
  Product2/1 -> Out3/1
  Product3/1 -> Out4/1
  Product4/1 -> Out5/1
  Product5/1 -> Out6/1
  Fault inject/1 -> Product5/1, Product4/1, Product3/1, Product2/1, Product1/1, Product/1

== system eVTOL_Small_nonandlin_algorithm_validation/各部件气动力和力矩/8组旋翼模块/FI-1-U15 ==
  FMxU1 : Inport
  FMyU1 : Inport  Port=2
  FMzU1 : Inport  Port=3
  MMxU1 : Inport  Port=4
  MMyU1 : Inport  Port=5
  MMzU1 : Inport  Port=6
  Fault inject : Inport  Port=7
  Product{,1..5} (6 alike) : Product
  Out1 : Outport
  Out2 : Outport  Port=2
  Out3 : Outport  Port=3
  Out4 : Outport  Port=4
  Out5 : Outport  Port=5
  Out6 : Outport  Port=6
  wires:
  FMxU1/1 -> Product/2
  FMyU1/1 -> Product1/2
  FMzU1/1 -> Product2/2
  MMxU1/1 -> Product3/2
  MMyU1/1 -> Product4/2
  MMzU1/1 -> Product5/2
  Product/1 -> Out1/1
  Product1/1 -> Out2/1
  Product2/1 -> Out3/1
  Product3/1 -> Out4/1
  Product4/1 -> Out5/1
  Product5/1 -> Out6/1
  Fault inject/1 -> Product5/1, Product4/1, Product3/1, Product2/1, Product1/1, Product/1

== system eVTOL_Small_nonandlin_algorithm_validation/各部件气动力和力矩/8组旋翼模块/FI-1-U2 ==
  Fault inject : Inport
  FMxU1 : Inport  Port=2
  FMyU1 : Inport  Port=3
  FMzU1 : Inport  Port=4
  MMxU1 : Inport  Port=5
  MMyU1 : Inport  Port=6
  MMzU1 : Inport  Port=7
  Product{,1..5} (6 alike) : Product
  Out1 : Outport
  Out2 : Outport  Port=2
  Out3 : Outport  Port=3
  Out4 : Outport  Port=4
  Out5 : Outport  Port=5
  Out6 : Outport  Port=6
  wires:
  FMxU1/1 -> Product/2
  FMyU1/1 -> Product1/2
  FMzU1/1 -> Product2/2
  MMxU1/1 -> Product3/2
  MMyU1/1 -> Product4/2
  MMzU1/1 -> Product5/2
  Product/1 -> Out1/1
  Product1/1 -> Out2/1
  Product2/1 -> Out3/1
  Product3/1 -> Out4/1
  Product4/1 -> Out5/1
  Product5/1 -> Out6/1
  Fault inject/1 -> Product5/1, Product4/1, Product3/1, Product2/1, Product1/1, Product/1

== system eVTOL_Small_nonandlin_algorithm_validation/各部件气动力和力矩/8组旋翼模块/FI-1-U3 ==
  FMxU1 : Inport
  FMyU1 : Inport  Port=2
  FMzU1 : Inport  Port=3
  MMxU1 : Inport  Port=4
  MMyU1 : Inport  Port=5
  MMzU1 : Inport  Port=6
  Fault inject : Inport  Port=7
  Product{,1..5} (6 alike) : Product
  Out1 : Outport
  Out2 : Outport  Port=2
  Out3 : Outport  Port=3
  Out4 : Outport  Port=4
  Out5 : Outport  Port=5
  Out6 : Outport  Port=6
  wires:
  FMxU1/1 -> Product/2
  FMyU1/1 -> Product1/2
  FMzU1/1 -> Product2/2
  MMxU1/1 -> Product3/2
  MMyU1/1 -> Product4/2
  MMzU1/1 -> Product5/2
  Product/1 -> Out1/1
  Product1/1 -> Out2/1
  Product2/1 -> Out3/1
  Product3/1 -> Out4/1
  Product4/1 -> Out5/1
  Product5/1 -> Out6/1
  Fault inject/1 -> Product5/1, Product4/1, Product3/1, Product2/1, Product1/1, Product/1

== system eVTOL_Small_nonandlin_algorithm_validation/各部件气动力和力矩/8组旋翼模块/FI-1-U4 ==
  Fault inject : Inport
  FMxU1 : Inport  Port=2
  FMyU1 : Inport  Port=3
  FMzU1 : Inport  Port=4
  MMxU1 : Inport  Port=5
  MMyU1 : Inport  Port=6
  MMzU1 : Inport  Port=7
  Product{,1..5} (6 alike) : Product
  Out1 : Outport
  Out2 : Outport  Port=2
  Out3 : Outport  Port=3
  Out4 : Outport  Port=4
  Out5 : Outport  Port=5
  Out6 : Outport  Port=6
  wires:
  FMxU1/1 -> Product/2
  FMyU1/1 -> Product1/2
  FMzU1/1 -> Product2/2
  MMxU1/1 -> Product3/2
  MMyU1/1 -> Product4/2
  MMzU1/1 -> Product5/2
  Product/1 -> Out1/1
  Product1/1 -> Out2/1
  Product2/1 -> Out3/1
  Product3/1 -> Out4/1
  Product4/1 -> Out5/1
  Product5/1 -> Out6/1
  Fault inject/1 -> Product5/1, Product4/1, Product3/1, Product2/1, Product1/1, Product/1

== system eVTOL_Small_nonandlin_algorithm_validation/各部件气动力和力矩/8组旋翼模块/FI-1-U5 ==
  FMxU1 : Inport
  FMyU1 : Inport  Port=2
  FMzU1 : Inport  Port=3
  MMxU1 : Inport  Port=4
  MMyU1 : Inport  Port=5
  MMzU1 : Inport  Port=6
  Fault inject : Inport  Port=7
  Product{,1..5} (6 alike) : Product
  Out1 : Outport
  Out2 : Outport  Port=2
  Out3 : Outport  Port=3
  Out4 : Outport  Port=4
  Out5 : Outport  Port=5
  Out6 : Outport  Port=6
  wires:
  FMxU1/1 -> Product/2
  FMyU1/1 -> Product1/2
  FMzU1/1 -> Product2/2
  MMxU1/1 -> Product3/2
  MMyU1/1 -> Product4/2
  MMzU1/1 -> Product5/2
  Product/1 -> Out1/1
  Product1/1 -> Out2/1
  Product2/1 -> Out3/1
  Product3/1 -> Out4/1
  Product4/1 -> Out5/1
  Product5/1 -> Out6/1
  Fault inject/1 -> Product5/1, Product4/1, Product3/1, Product2/1, Product1/1, Product/1

== system eVTOL_Small_nonandlin_algorithm_validation/各部件气动力和力矩/8组旋翼模块/FI-1-U6 ==
  Fault inject : Inport
  FMxU1 : Inport  Port=2
  FMyU1 : Inport  Port=3
  FMzU1 : Inport  Port=4
  MMxU1 : Inport  Port=5
  MMyU1 : Inport  Port=6
  MMzU1 : Inport  Port=7
  Product{,1..5} (6 alike) : Product
  Out1 : Outport
  Out2 : Outport  Port=2
  Out3 : Outport  Port=3
  Out4 : Outport  Port=4
  Out5 : Outport  Port=5
  Out6 : Outport  Port=6
  wires:
  FMxU1/1 -> Product/2
  FMyU1/1 -> Product1/2
  FMzU1/1 -> Product2/2
  MMxU1/1 -> Product3/2
  MMyU1/1 -> Product4/2
  MMzU1/1 -> Product5/2
  Product/1 -> Out1/1
  Product1/1 -> Out2/1
  Product2/1 -> Out3/1
  Product3/1 -> Out4/1
  Product4/1 -> Out5/1
  Product5/1 -> Out6/1
  Fault inject/1 -> Product5/1, Product4/1, Product3/1, Product2/1, Product1/1, Product/1

== system eVTOL_Small_nonandlin_algorithm_validation/各部件气动力和力矩/8组旋翼模块/FI-1-U7 ==
  FMxU1 : Inport
  FMyU1 : Inport  Port=2
  FMzU1 : Inport  Port=3
  MMxU1 : Inport  Port=4
  MMyU1 : Inport  Port=5
  MMzU1 : Inport  Port=6
  Fault inject : Inport  Port=7
  Product{,1..5} (6 alike) : Product
  Out1 : Outport
  Out2 : Outport  Port=2
  Out3 : Outport  Port=3
  Out4 : Outport  Port=4
  Out5 : Outport  Port=5
  Out6 : Outport  Port=6
  wires:
  FMxU1/1 -> Product/2
  FMyU1/1 -> Product1/2
  FMzU1/1 -> Product2/2
  MMxU1/1 -> Product3/2
  MMyU1/1 -> Product4/2
  MMzU1/1 -> Product5/2
  Product/1 -> Out1/1
  Product1/1 -> Out2/1
  Product2/1 -> Out3/1
  Product3/1 -> Out4/1
  Product4/1 -> Out5/1
  Product5/1 -> Out6/1
  Fault inject/1 -> Product5/1, Product4/1, Product3/1, Product2/1, Product1/1, Product/1

== system eVTOL_Small_nonandlin_algorithm_validation/各部件气动力和力矩/8组旋翼模块/FI-1-U8 ==
  Fault inject : Inport
  FMxU1 : Inport  Port=2
  FMyU1 : Inport  Port=3
  FMzU1 : Inport  Port=4
  MMxU1 : Inport  Port=5
  MMyU1 : Inport  Port=6
  MMzU1 : Inport  Port=7
  Product{,1..5} (6 alike) : Product
  Out1 : Outport
  Out2 : Outport  Port=2
  Out3 : Outport  Port=3
  Out4 : Outport  Port=4
  Out5 : Outport  Port=5
  Out6 : Outport  Port=6
  wires:
  FMxU1/1 -> Product/2
  FMyU1/1 -> Product1/2
  FMzU1/1 -> Product2/2
  MMxU1/1 -> Product3/2
  MMyU1/1 -> Product4/2
  MMzU1/1 -> Product5/2
  Product/1 -> Out1/1
  Product1/1 -> Out2/1
  Product2/1 -> Out3/1
  Product3/1 -> Out4/1
  Product4/1 -> Out5/1
  Product5/1 -> Out6/1
  Fault inject/1 -> Product5/1, Product4/1, Product3/1, Product2/1, Product1/1, Product/1

== system eVTOL_Small_nonandlin_algorithm_validation/各部件气动力和力矩/8组旋翼模块/FI-1-U9 ==
  FMxU1 : Inport
  FMyU1 : Inport  Port=2
  FMzU1 : Inport  Port=3
  MMxU1 : Inport  Port=4
  MMyU1 : Inport  Port=5
  MMzU1 : Inport  Port=6
  Fault inject : Inport  Port=7
  Product{,1..5} (6 alike) : Product
  Out1 : Outport
  Out2 : Outport  Port=2
  Out3 : Outport  Port=3
  Out4 : Outport  Port=4
  Out5 : Outport  Port=5
  Out6 : Outport  Port=6
  wires:
  FMxU1/1 -> Product/2
  FMyU1/1 -> Product1/2
  FMzU1/1 -> Product2/2
  MMxU1/1 -> Product3/2
  MMyU1/1 -> Product4/2
  MMzU1/1 -> Product5/2
  Product/1 -> Out1/1
  Product1/1 -> Out2/1
  Product2/1 -> Out3/1
  Product3/1 -> Out4/1
  Product4/1 -> Out5/1
  Product5/1 -> Out6/1
  Fault inject/1 -> Product5/1, Product4/1, Product3/1, Product2/1, Product1/1, Product/1

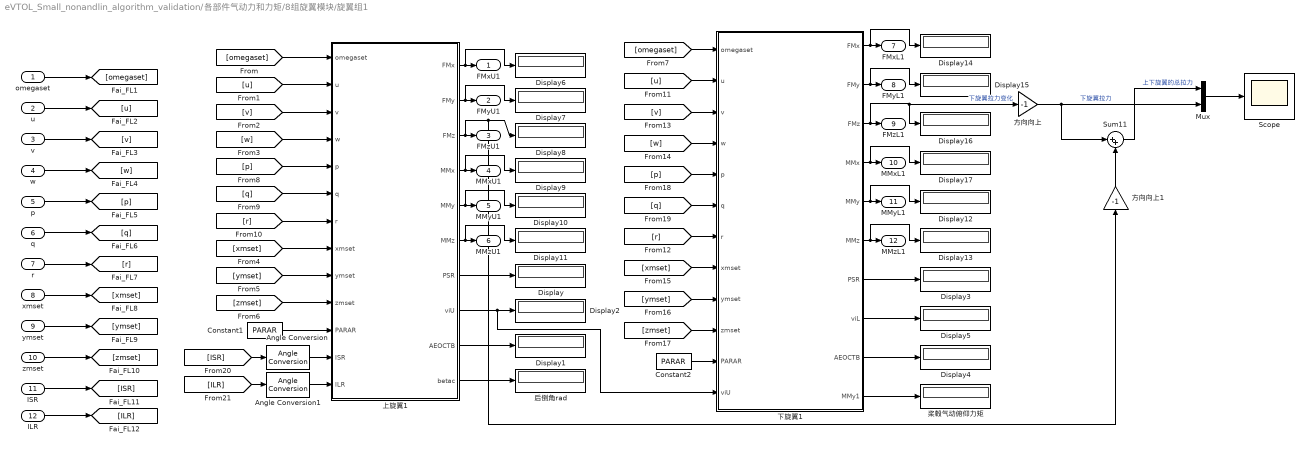
== system eVTOL_Small_nonandlin_algorithm_validation/各部件气动力和力矩/8组旋翼模块/旋翼组1 ==
  omegaset : Inport
  u : Inport  Port=2
  v : Inport  Port=3
  w : Inport  Port=4
  p : Inport  Port=5
  q : Inport  Port=6
  r : Inport  Port=7
  xmset : Inport  Port=8
  ymset : Inport  Port=9
  zmset : Inport  Port=10
  ISR : Inport  Port=11
  ILR : Inport  Port=12
  Angle Conversion : aerolibconvert2/Angle Conversion  IU=deg  OU=rad
  Angle Conversion1 : aerolibconvert2/Angle Conversion  IU=deg  OU=rad
  Constant1 : Constant  Value=PARAR
  Constant2 : Constant  Value=PARAR
  Display{,1..17} (18 alike) : Display
  Mux : Mux  Inputs=2
  Scope : Scope
  Sum11 : Sum  Inputs=|++
  上旋翼1 : MATLAB Function  TreatAsAtomicUnit=on
  下旋翼1 : MATLAB Function  TreatAsAtomicUnit=on
  后倒角rad : Display
  方向向上 : Gain  Gain=-1
  方向向上1 : Gain  Gain=-1
  桨毂气动俯仰力矩 : Display
  FMxU1 : Outport  VectorParamsAs1DForOutWhenUnconnected=off
  FMyU1 : Outport  Port=2  VectorParamsAs1DForOutWhenUnconnected=off
  FMzU1 : Outport  Port=3  VectorParamsAs1DForOutWhenUnconnected=off
  MMxU1 : Outport  Port=4  VectorParamsAs1DForOutWhenUnconnected=off
  MMyU1 : Outport  Port=5  VectorParamsAs1DForOutWhenUnconnected=off
  MMzU1 : Outport  Port=6  VectorParamsAs1DForOutWhenUnconnected=off
  FMxL1 : Outport  Port=7  VectorParamsAs1DForOutWhenUnconnected=off
  FMyL1 : Outport  Port=8  VectorParamsAs1DForOutWhenUnconnected=off
  FMzL1 : Outport  Port=9  VectorParamsAs1DForOutWhenUnconnected=off
  MMxL1 : Outport  Port=10  VectorParamsAs1DForOutWhenUnconnected=off
  MMyL1 : Outport  Port=11  VectorParamsAs1DForOutWhenUnconnected=off
  MMzL1 : Outport  Port=12  VectorParamsAs1DForOutWhenUnconnected=off
  wires:
  [omegaset] -> 上旋翼1/1(omegaset)
  [u] -> 上旋翼1/2(u)
  [v] -> 上旋翼1/3(v)
  [w] -> 上旋翼1/4(w)
  omegaset/1 -> [omegaset]
  u/1 -> [u]
  v/1 -> [v]
  w/1 -> [w]
  p/1 -> [p]
  r/1 -> [r]
  q/1 -> [q]
  [p] -> 上旋翼1/5(p)
  [q] -> 上旋翼1/6(q)
  [r] -> 上旋翼1/7(r)
  xmset/1 -> [xmset]
  ymset/1 -> [ymset]
  zmset/1 -> [zmset]
  [xmset] -> 上旋翼1/8(xmset)
  [ymset] -> 上旋翼1/9(ymset)
  [zmset] -> 上旋翼1/10(zmset)
  上旋翼1/1(FMx) -> Display6/1, FMxU1/1
  上旋翼1/2(FMy) -> Display7/1, FMyU1/1
  上旋翼1/4(MMx) -> Display9/1, MMxU1/1
  上旋翼1/5(MMy) -> Display10/1, MMyU1/1
  上旋翼1/6(MMz) -> Display11/1, MMzU1/1
  上旋翼1/7(PSR) -> Display/1
  上旋翼1/9(AEOCTB) -> Display1/1
  上旋翼1/8(viU) -> 下旋翼1/12(viU), Display2/1
  下旋翼1/9(AEOCTB) -> Display4/1
  下旋翼1/2(FMy) -> Display15/1, FMyL1/1
  下旋翼1/1(FMx) -> Display14/1, FMxL1/1
  下旋翼1/8(viL) -> Display5/1
  下旋翼1/7(PSR) -> Display3/1
  下旋翼1/6(MMz) -> Display13/1, MMzL1/1
  下旋翼1/4(MMx) -> Display17/1, MMxL1/1
  下旋翼1/5(MMy) -> Display12/1, MMyL1/1
  [p] -> 下旋翼1/5(p)
  [r] -> 下旋翼1/7(r)
  [xmset] -> 下旋翼1/8(xmset)
  [zmset] -> 下旋翼1/10(zmset)
  [v] -> 下旋翼1/3(v)
  [ymset] -> 下旋翼1/9(ymset)
  [q] -> 下旋翼1/6(q)
  [w] -> 下旋翼1/4(w)
  [omegaset] -> 下旋翼1/1(omegaset)
  [u] -> 下旋翼1/2(u)
  Constant1/1 -> 上旋翼1/11(PARAR)
  Constant2/1 -> 下旋翼1/11(PARAR)
  上旋翼1/10(betac) -> 后倒角rad/1
  下旋翼1/10(MMy1) -> 桨毂气动俯仰力矩/1
  ISR/1 -> [ISR]
  ILR/1 -> [ILR]
  [ISR] -> Angle Conversion/1
  [ILR] -> Angle Conversion1/1
  Angle Conversion/1 -> 上旋翼1/12(ISR)
  Angle Conversion1/1 -> 上旋翼1/13(ILR)
  下旋翼1/3(FMz) -> Display16/1, 方向向上/1, FMzL1/1  "下旋翼拉力变化"
  方向向上1/1 -> Sum11/2
  Mux/1 -> Scope/1
  上旋翼1/3(FMz) -> 方向向上1/1, Display8/1, FMzU1/1
  方向向上/1 -> Sum11/1, Mux/2  "下旋翼拉力"
  Sum11/1 -> Mux/1  "上下旋翼的总拉力"

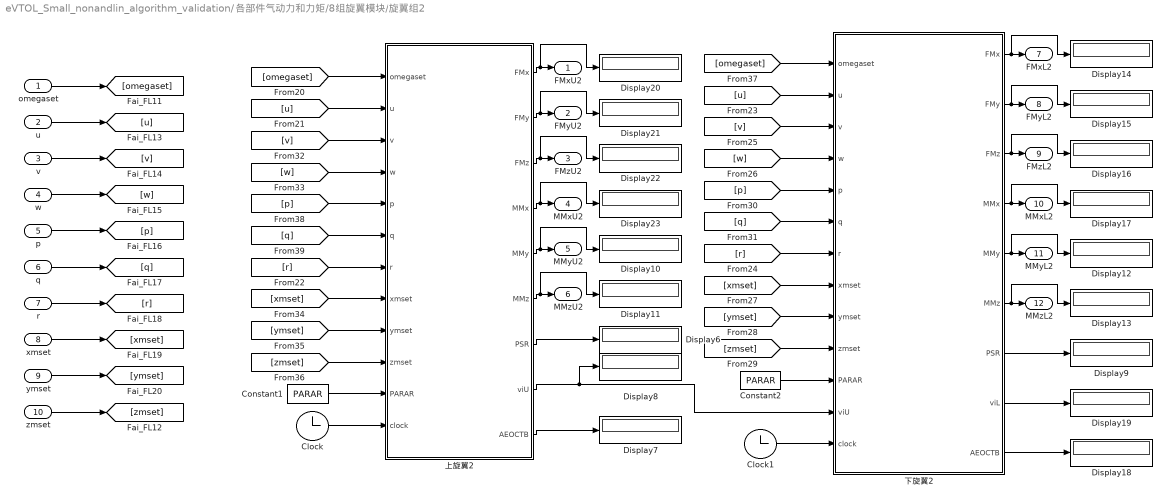
== system eVTOL_Small_nonandlin_algorithm_validation/各部件气动力和力矩/8组旋翼模块/旋翼组2 ==
  omegaset : Inport
  u : Inport  Port=2
  v : Inport  Port=3
  w : Inport  Port=4
  p : Inport  Port=5
  q : Inport  Port=6
  r : Inport  Port=7
  xmset : Inport  Port=8
  ymset : Inport  Port=9
  zmset : Inport  Port=10
  Clock : Clock
  Clock1 : Clock
  Constant1 : Constant  Value=PARAR
  Constant2 : Constant  Value=PARAR
  Display{6..23} (18 alike) : Display
  上旋翼2 : MATLAB Function  TreatAsAtomicUnit=on
  下旋翼2 : MATLAB Function  TreatAsAtomicUnit=on
  FMxU2 : Outport  VectorParamsAs1DForOutWhenUnconnected=off
  FMyU2 : Outport  Port=2  VectorParamsAs1DForOutWhenUnconnected=off
  FMzU2 : Outport  Port=3  VectorParamsAs1DForOutWhenUnconnected=off
  MMxU2 : Outport  Port=4  VectorParamsAs1DForOutWhenUnconnected=off
  MMyU2 : Outport  Port=5  VectorParamsAs1DForOutWhenUnconnected=off
  MMzU2 : Outport  Port=6  VectorParamsAs1DForOutWhenUnconnected=off
  FMxL2 : Outport  Port=7  VectorParamsAs1DForOutWhenUnconnected=off
  FMyL2 : Outport  Port=8  VectorParamsAs1DForOutWhenUnconnected=off
  FMzL2 : Outport  Port=9  VectorParamsAs1DForOutWhenUnconnected=off
  MMxL2 : Outport  Port=10  VectorParamsAs1DForOutWhenUnconnected=off
  MMyL2 : Outport  Port=11  VectorParamsAs1DForOutWhenUnconnected=off
  MMzL2 : Outport  Port=12  VectorParamsAs1DForOutWhenUnconnected=off
  wires:
  [u] -> 下旋翼2/2(u)
  [u] -> 上旋翼2/2(u)
  下旋翼2/4(MMx) -> Display17/1, MMxL2/1
  [w] -> 下旋翼2/4(w)
  上旋翼2/7(PSR) -> Display6/1
  [p] -> 下旋翼2/5(p)
  [omegaset] -> 下旋翼2/1(omegaset)
  [r] -> 上旋翼2/7(r)
  下旋翼2/6(MMz) -> Display13/1, MMzL2/1
  [q] -> 下旋翼2/6(q)
  下旋翼2/1(FMx) -> Display14/1, FMxL2/1
  r/1 -> [r]
  [zmset] -> 下旋翼2/10(zmset)
  [w] -> 上旋翼2/4(w)
  [r] -> 下旋翼2/7(r)
  下旋翼2/2(FMy) -> Display15/1, FMyL2/1
  [ymset] -> 下旋翼2/9(ymset)
  [v] -> 下旋翼2/3(v)
  上旋翼2/9(AEOCTB) -> Display7/1
  上旋翼2/5(MMy) -> Display10/1, MMyU2/1
  下旋翼2/5(MMy) -> Display12/1, MMyL2/1
  zmset/1 -> [zmset]
  [ymset] -> 上旋翼2/9(ymset)
  上旋翼2/3(FMz) -> Display22/1, FMzU2/1
  上旋翼2/6(MMz) -> Display11/1, MMzU2/1
  下旋翼2/3(FMz) -> Display16/1, FMzL2/1
  [xmset] -> 上旋翼2/8(xmset)
  [zmset] -> 上旋翼2/10(zmset)
  [xmset] -> 下旋翼2/8(xmset)
  上旋翼2/2(FMy) -> Display21/1, FMyU2/1
  [omegaset] -> 上旋翼2/1(omegaset)
  omegaset/1 -> [omegaset]
  xmset/1 -> [xmset]
  下旋翼2/8(viL) -> Display19/1
  [q] -> 上旋翼2/6(q)
  q/1 -> [q]
  [p] -> 上旋翼2/5(p)
  ymset/1 -> [ymset]
  p/1 -> [p]
  w/1 -> [w]
  上旋翼2/1(FMx) -> Display20/1, FMxU2/1
  v/1 -> [v]
  下旋翼2/7(PSR) -> Display9/1
  下旋翼2/9(AEOCTB) -> Display18/1
  上旋翼2/4(MMx) -> Display23/1, MMxU2/1
  u/1 -> [u]
  [v] -> 上旋翼2/3(v)
  上旋翼2/8(viU) -> Display8/1, 下旋翼2/12(viU)
  Constant1/1 -> 上旋翼2/11(PARAR)
  Constant2/1 -> 下旋翼2/11(PARAR)
  Clock/1 -> 上旋翼2/12(clock)
  Clock1/1 -> 下旋翼2/13(clock)

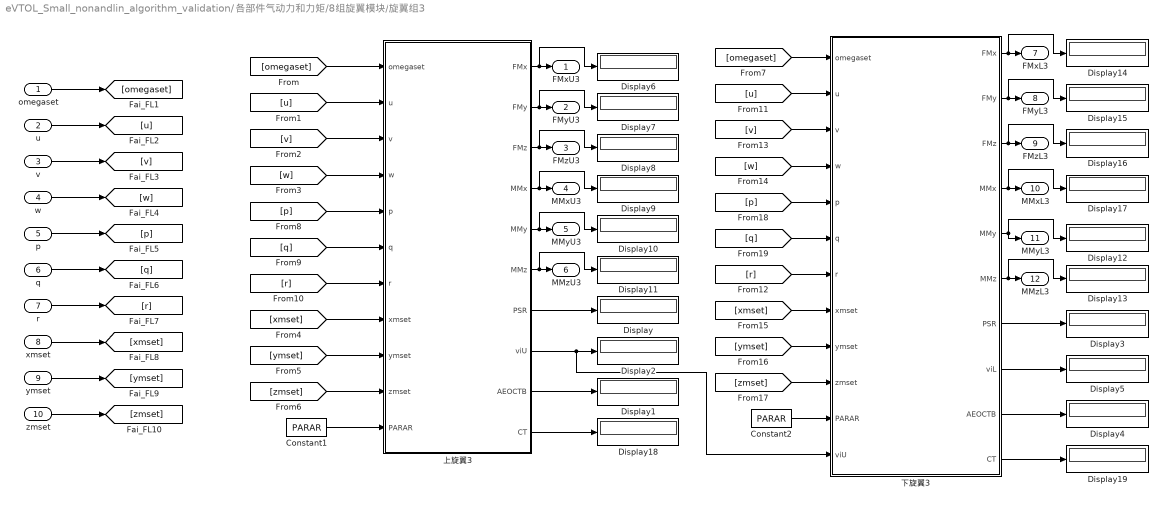
== system eVTOL_Small_nonandlin_algorithm_validation/各部件气动力和力矩/8组旋翼模块/旋翼组3 ==
  omegaset : Inport
  u : Inport  Port=2
  v : Inport  Port=3
  w : Inport  Port=4
  p : Inport  Port=5
  q : Inport  Port=6
  r : Inport  Port=7
  xmset : Inport  Port=8
  ymset : Inport  Port=9
  zmset : Inport  Port=10
  Constant1 : Constant  Value=PARAR
  Constant2 : Constant  Value=PARAR
  Display{,1..19} (20 alike) : Display
  上旋翼3 : MATLAB Function  TreatAsAtomicUnit=on
  下旋翼3 : MATLAB Function  TreatAsAtomicUnit=on
  FMxU3 : Outport  VectorParamsAs1DForOutWhenUnconnected=off
  FMyU3 : Outport  Port=2  VectorParamsAs1DForOutWhenUnconnected=off
  FMzU3 : Outport  Port=3  VectorParamsAs1DForOutWhenUnconnected=off
  MMxU3 : Outport  Port=4  VectorParamsAs1DForOutWhenUnconnected=off
  MMyU3 : Outport  Port=5  VectorParamsAs1DForOutWhenUnconnected=off
  MMzU3 : Outport  Port=6  VectorParamsAs1DForOutWhenUnconnected=off
  FMxL3 : Outport  Port=7  VectorParamsAs1DForOutWhenUnconnected=off
  FMyL3 : Outport  Port=8  VectorParamsAs1DForOutWhenUnconnected=off
  FMzL3 : Outport  Port=9  VectorParamsAs1DForOutWhenUnconnected=off
  MMxL3 : Outport  Port=10  VectorParamsAs1DForOutWhenUnconnected=off
  MMyL3 : Outport  Port=11  VectorParamsAs1DForOutWhenUnconnected=off
  MMzL3 : Outport  Port=12  VectorParamsAs1DForOutWhenUnconnected=off
  wires:
  [omegaset] -> 上旋翼3/1(omegaset)
  [u] -> 上旋翼3/2(u)
  [v] -> 上旋翼3/3(v)
  [w] -> 上旋翼3/4(w)
  omegaset/1 -> [omegaset]
  u/1 -> [u]
  v/1 -> [v]
  w/1 -> [w]
  p/1 -> [p]
  r/1 -> [r]
  q/1 -> [q]
  [p] -> 上旋翼3/5(p)
  [q] -> 上旋翼3/6(q)
  [r] -> 上旋翼3/7(r)
  xmset/1 -> [xmset]
  ymset/1 -> [ymset]
  zmset/1 -> [zmset]
  [xmset] -> 上旋翼3/8(xmset)
  [ymset] -> 上旋翼3/9(ymset)
  [zmset] -> 上旋翼3/10(zmset)
  上旋翼3/1(FMx) -> Display6/1, FMxU3/1
  上旋翼3/2(FMy) -> Display7/1, FMyU3/1
  上旋翼3/3(FMz) -> Display8/1, FMzU3/1
  上旋翼3/4(MMx) -> Display9/1, MMxU3/1
  上旋翼3/5(MMy) -> Display10/1, MMyU3/1
  上旋翼3/6(MMz) -> Display11/1, MMzU3/1
  上旋翼3/7(PSR) -> Display/1
  上旋翼3/9(AEOCTB) -> Display1/1
  上旋翼3/8(viU) -> 下旋翼3/12(viU), Display2/1
  下旋翼3/9(AEOCTB) -> Display4/1
  下旋翼3/3(FMz) -> Display16/1, FMzL3/1
  下旋翼3/2(FMy) -> Display15/1, FMyL3/1
  下旋翼3/1(FMx) -> Display14/1, FMxL3/1
  下旋翼3/8(viL) -> Display5/1
  下旋翼3/7(PSR) -> Display3/1
  下旋翼3/6(MMz) -> Display13/1, MMzL3/1
  下旋翼3/4(MMx) -> Display17/1, MMxL3/1
  下旋翼3/5(MMy) -> MMyL3/1, Display12/1
  [p] -> 下旋翼3/5(p)
  [r] -> 下旋翼3/7(r)
  [xmset] -> 下旋翼3/8(xmset)
  [zmset] -> 下旋翼3/10(zmset)
  [v] -> 下旋翼3/3(v)
  [ymset] -> 下旋翼3/9(ymset)
  [q] -> 下旋翼3/6(q)
  [w] -> 下旋翼3/4(w)
  [omegaset] -> 下旋翼3/1(omegaset)
  [u] -> 下旋翼3/2(u)
  Constant1/1 -> 上旋翼3/11(PARAR)
  Constant2/1 -> 下旋翼3/11(PARAR)
  上旋翼3/10(CT) -> Display18/1
  下旋翼3/10(CT) -> Display19/1

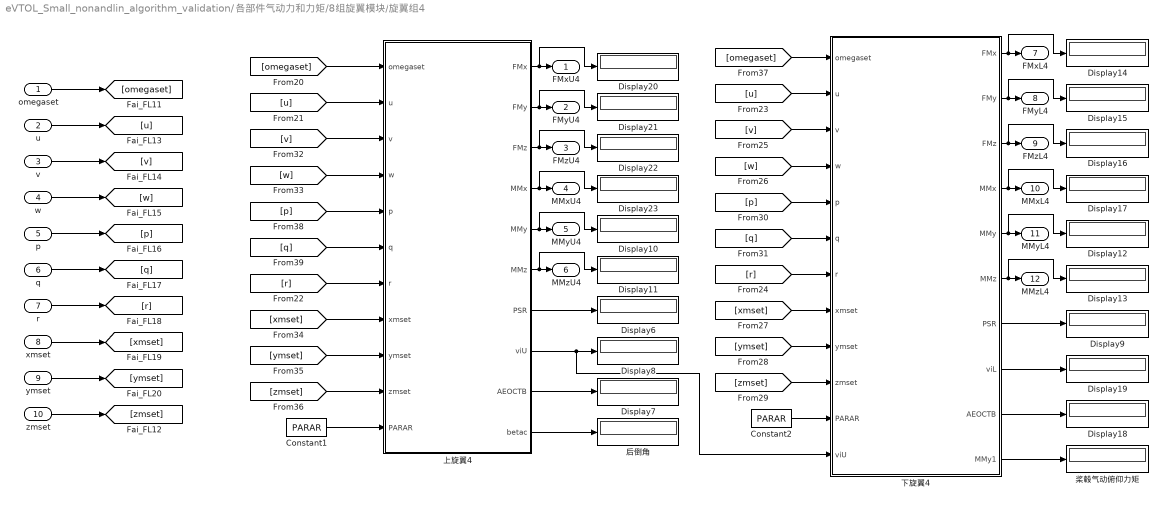
== system eVTOL_Small_nonandlin_algorithm_validation/各部件气动力和力矩/8组旋翼模块/旋翼组4 ==
  omegaset : Inport
  u : Inport  Port=2
  v : Inport  Port=3
  w : Inport  Port=4
  p : Inport  Port=5
  q : Inport  Port=6
  r : Inport  Port=7
  xmset : Inport  Port=8
  ymset : Inport  Port=9
  zmset : Inport  Port=10
  Constant1 : Constant  Value=PARAR
  Constant2 : Constant  Value=PARAR
  Display{6..23} (18 alike) : Display
  上旋翼4 : MATLAB Function  TreatAsAtomicUnit=on
  下旋翼4 : MATLAB Function  TreatAsAtomicUnit=on
  后倒角 : Display
  桨毂气动俯仰力矩 : Display
  FMxU4 : Outport  VectorParamsAs1DForOutWhenUnconnected=off
  FMyU4 : Outport  Port=2  VectorParamsAs1DForOutWhenUnconnected=off
  FMzU4 : Outport  Port=3  VectorParamsAs1DForOutWhenUnconnected=off
  MMxU4 : Outport  Port=4  VectorParamsAs1DForOutWhenUnconnected=off
  MMyU4 : Outport  Port=5  VectorParamsAs1DForOutWhenUnconnected=off
  MMzU4 : Outport  Port=6  VectorParamsAs1DForOutWhenUnconnected=off
  FMxL4 : Outport  Port=7  VectorParamsAs1DForOutWhenUnconnected=off
  FMyL4 : Outport  Port=8  VectorParamsAs1DForOutWhenUnconnected=off
  FMzL4 : Outport  Port=9  VectorParamsAs1DForOutWhenUnconnected=off
  MMxL4 : Outport  Port=10  VectorParamsAs1DForOutWhenUnconnected=off
  MMyL4 : Outport  Port=11  VectorParamsAs1DForOutWhenUnconnected=off
  MMzL4 : Outport  Port=12  VectorParamsAs1DForOutWhenUnconnected=off
  wires:
  [u] -> 下旋翼4/2(u)
  [u] -> 上旋翼4/2(u)
  下旋翼4/4(MMx) -> Display17/1, MMxL4/1
  [w] -> 下旋翼4/4(w)
  上旋翼4/7(PSR) -> Display6/1
  [p] -> 下旋翼4/5(p)
  [omegaset] -> 下旋翼4/1(omegaset)
  [r] -> 上旋翼4/7(r)
  下旋翼4/6(MMz) -> Display13/1, MMzL4/1
  [q] -> 下旋翼4/6(q)
  下旋翼4/1(FMx) -> Display14/1, FMxL4/1
  r/1 -> [r]
  [zmset] -> 下旋翼4/10(zmset)
  [w] -> 上旋翼4/4(w)
  [r] -> 下旋翼4/7(r)
  下旋翼4/2(FMy) -> Display15/1, FMyL4/1
  [ymset] -> 下旋翼4/9(ymset)
  [v] -> 下旋翼4/3(v)
  上旋翼4/9(AEOCTB) -> Display7/1
  上旋翼4/5(MMy) -> Display10/1, MMyU4/1
  下旋翼4/5(MMy) -> Display12/1, MMyL4/1
  zmset/1 -> [zmset]
  [ymset] -> 上旋翼4/9(ymset)
  上旋翼4/3(FMz) -> Display22/1, FMzU4/1
  上旋翼4/6(MMz) -> Display11/1, MMzU4/1
  下旋翼4/3(FMz) -> Display16/1, FMzL4/1
  [xmset] -> 上旋翼4/8(xmset)
  [zmset] -> 上旋翼4/10(zmset)
  [xmset] -> 下旋翼4/8(xmset)
  上旋翼4/2(FMy) -> Display21/1, FMyU4/1
  [omegaset] -> 上旋翼4/1(omegaset)
  omegaset/1 -> [omegaset]
  xmset/1 -> [xmset]
  下旋翼4/8(viL) -> Display19/1
  [q] -> 上旋翼4/6(q)
  q/1 -> [q]
  [p] -> 上旋翼4/5(p)
  ymset/1 -> [ymset]
  p/1 -> [p]
  w/1 -> [w]
  上旋翼4/1(FMx) -> Display20/1, FMxU4/1
  v/1 -> [v]
  下旋翼4/7(PSR) -> Display9/1
  下旋翼4/9(AEOCTB) -> Display18/1
  上旋翼4/4(MMx) -> Display23/1, MMxU4/1
  u/1 -> [u]
  [v] -> 上旋翼4/3(v)
  上旋翼4/8(viU) -> 下旋翼4/12(viU), Display8/1
  Constant1/1 -> 上旋翼4/11(PARAR)
  Constant2/1 -> 下旋翼4/11(PARAR)
  上旋翼4/10(betac) -> 后倒角/1
  下旋翼4/10(MMy1) -> 桨毂气动俯仰力矩/1
